simulink model "threephasePWMinverter"  (R2014a)
settings: Solver=ode45  StartTime=0.0  StopTime=0.1  RelTol=1e-3
libraries: powerlib x12, powerlib_meascontrol x2
settings Model: Creator=Dell  LastModifiedBy=Dell

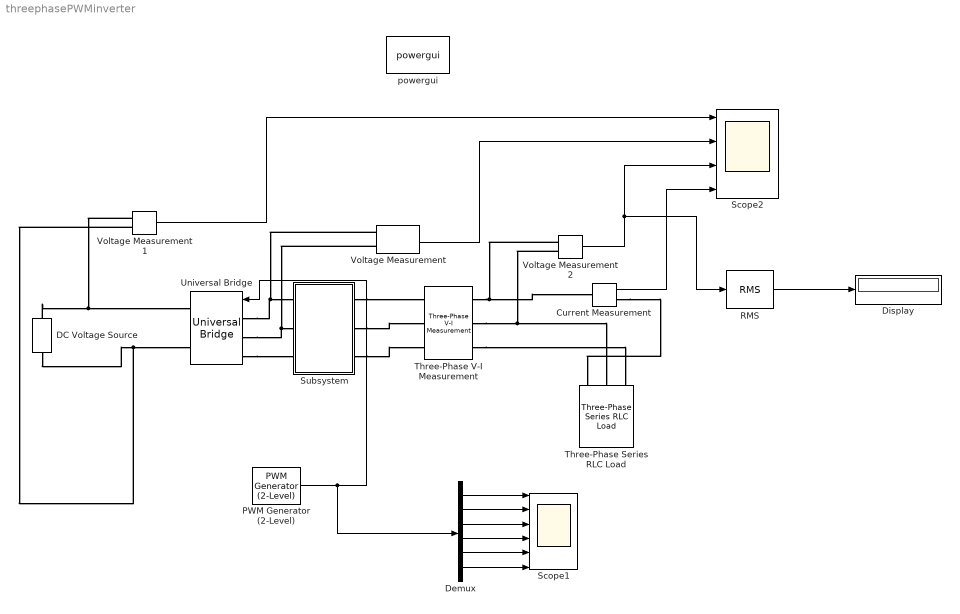
== system threephasePWMinverter ==
  Current Measurement : powerlib/Measurements/Current Measurement  PhasorSimulation=off  OutputType=Complex  PSBequivalent=0
  DC Voltage Source : powerlib/Electrical Sources/DC Voltage Source  Amplitude=500  Measurements=None
  Demux : Demux  Outputs=6
  Display : Display
  PWM Generator (2-Level) : powerlib_meascontrol/Pulse & Signal Generators/PWM Generator (2-Level)  ModulatorType=Three-phase bridge (6 pulses)  ModulatorMode=Unsynchronized  nF=27  Fc=3000  ModulatingSignals=on  m=0.8  Freq=50  Phase=0  Ts=1e-6
  RMS : powerlib_meascontrol/Measurements/RMS  TrueRMS=on  Freq=50  RMSInit=100  Ts=1e-6
  Scope1 : Scope  NumInputPorts=6
      settings: TimeRange=0.1  YMin=-5~-5~-5~-5~-5~-5  YMax=5~5~5~5~5~5
  Scope2 : Scope  NumInputPorts=4
      settings: YMin=380~-500~-400~-25  YMax=420~500~400~25  SaveName=ScopeData2
  Subsystem : Subsystem
  Three-Phase Series RLC Load : powerlib/Elements/Three-Phase Series RLC Load  LConnTagsString=A|B|C  Configuration=Y (grounded)  NominalVoltage=400  NominalFrequency=50  ActivePower=20e3  InductivePower=0  CapacitivePower=0  Measurements=None  LoadType=constant Z
  Three-Phase V-I Measurement : powerlib/Measurements/Three-Phase V-I Measurement  VoltageMeasurement=phase-to-ground  SetLabelV=on  LabelV=Vabc  Vpu=off  VpuLL=off  CurrentMeasurement=yes  SetLabelI=on  LabelI=Iabc  Ipu=off  Pbase=100e6  Vbase=500e3  OutputType=Complex  PhasorSimulation=off  PSBequivalent=0
  Universal Bridge : powerlib/Power Electronics/Universal Bridge  Arms=3  SnubberResistance=1e5  SnubberCapacitance=inf  Device=IGBT / Diodes  Ron=1e-3  Lon=0  ForwardVoltages="[  0  0  ]"  ForwardVoltage=0  GTOparameters=[ 10e-6 , 20e-6 ]  IGBTparameters=[ 1e-6 , 2e-6 ]  Measurements=None  Measurements_2=None  converterType=Rectifier
  Voltage Measurement : powerlib/Measurements/Voltage Measurement  PhasorSimulation=off  OutputType=Complex  PSBequivalent=0
  Voltage Measurement1 : powerlib/Measurements/Voltage Measurement  PhasorSimulation=off  OutputType=Complex  PSBequivalent=0
  Voltage Measurement2 : powerlib/Measurements/Voltage Measurement  PhasorSimulation=off  OutputType=Complex  PSBequivalent=0
  powergui : powerlib/powergui  Priority=1  SimulationMode=Continuous  SolverType=Tustin  SampleTime=1e-6  frequency=60  SPID=off  DisableSnubberDevices=off  DisableRonSwitches=off  DisableVfSwitches=off  SwTol=0  Interpol=off  DisplayEquations=off  Ts=0  methode=off  frequencyindice=0  Pbase=100e6  ErrMax=1e-4  Iterations=50  UnitsV=kV  UnitsW=MW  FunctionMessages=off  echomessages=off  HookPort=off  EnableUseOfTLC=off  x0status=blocks  RestoreLinks=warning  ResistiveCurrentMeasurement=off  Frange=[0:2:500]  Ylog=off  Xlog=on  ShowGrid=off  save=off  variable=ZData  structure=0  ZoomFFT=off  StartTime=0.0  cycles=1  DisplayStyle=1  fundamental=60  FreqAxis=off  MaxFrequency=1000  frequencyindicesteady=1  RmsSteady=1  display=off
  wires:
  Current Measurement/1 -> Scope2/4
  Voltage Measurement2/1 -> RMS/1, Scope2/3
  Voltage Measurement/1 -> Scope2/2
  Voltage Measurement1/1 -> Scope2/1
  RMS/1 -> Display/1
  PWM Generator (2-Level)/1 -> Demux/1, Universal Bridge/1
  Demux/1 -> Scope1/1
  Demux/2 -> Scope1/2
  Demux/3 -> Scope1/3
  Demux/4 -> Scope1/4
  Demux/5 -> Scope1/5
  Demux/6 -> Scope1/6
  connections:
  DC Voltage Source/RConn1 -- Voltage Measurement1/LConn1 -- Universal Bridge/RConn1
  DC Voltage Source/LConn1 -- Voltage Measurement1/LConn2 -- Universal Bridge/RConn2
  Universal Bridge/LConn1 -- Voltage Measurement/LConn1 -- Subsystem/LConn1
  Universal Bridge/LConn2 -- Voltage Measurement/LConn2 -- Subsystem/LConn2
  Universal Bridge/LConn3 -- Subsystem/LConn3
  Subsystem/RConn1 -- Three-Phase V-I Measurement/LConn1
  Subsystem/RConn2 -- Three-Phase V-I Measurement/LConn2
  Subsystem/RConn3 -- Three-Phase V-I Measurement/LConn3
  Three-Phase V-I Measurement/RConn1 -- Voltage Measurement2/LConn1 -- Current Measurement/LConn1
  Three-Phase V-I Measurement/RConn2 -- Voltage Measurement2/LConn2 -- Three-Phase Series RLC Load/LConn2
  Three-Phase V-I Measurement/RConn3 -- Three-Phase Series RLC Load/LConn3
  Current Measurement/RConn1 -- Three-Phase Series RLC Load/LConn1

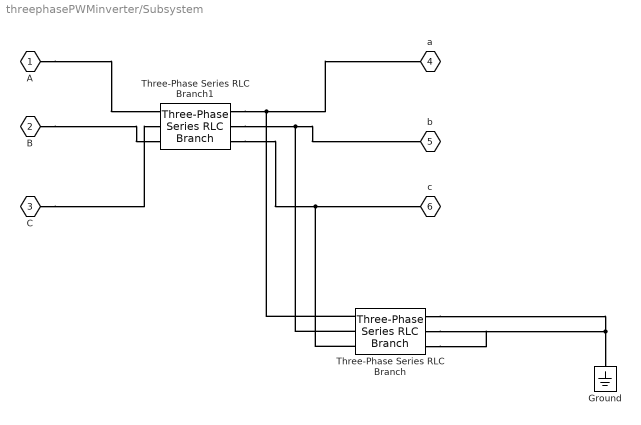
== system threephasePWMinverter/Subsystem ==
  Ground : powerlib/Elements/Ground  LConnTagsString=a
  Three-Phase Series RLC Branch : powerlib/Elements/Three-Phase Series RLC Branch  LConnTagsString=A|B|C  RConnTagsString=A|B|C  BranchType=C  Resistance=1  Inductance=1e-3  Capacitance=480e-6  Measurements=None
  Three-Phase Series RLC Branch1 : powerlib/Elements/Three-Phase Series RLC Branch  LConnTagsString=A|B|C  RConnTagsString=A|B|C  BranchType=L  Resistance=1  Inductance=22e-3  Capacitance=1e-6  Measurements=None
  A : PMIOPort  Port=1  Side=Left
  B : PMIOPort  Port=2  Side=Left
  C : PMIOPort  Port=3  Side=Left
  a : PMIOPort  Port=4  Side=Right
  b : PMIOPort  Port=5  Side=Right
  c : PMIOPort  Port=6  Side=Right
  connections:
  A/RConn1 -- Three-Phase Series RLC Branch1/LConn1
  B/RConn1 -- Three-Phase Series RLC Branch1/LConn3
  C/RConn1 -- Three-Phase Series RLC Branch1/LConn2
  Three-Phase Series RLC Branch1/RConn1 -- Three-Phase Series RLC Branch/LConn1 -- a/RConn1
  Three-Phase Series RLC Branch1/RConn2 -- Three-Phase Series RLC Branch/LConn2 -- b/RConn1
  Three-Phase Series RLC Branch1/RConn3 -- Three-Phase Series RLC Branch/LConn3 -- c/RConn1
  Three-Phase Series RLC Branch/RConn1 -- Three-Phase Series RLC Branch/RConn3 -- Three-Phase Series RLC Branch/RConn2 -- Ground/LConn1
